simulink model "robotarm_A12"  (R2018b)
settings: Solver=FixedStepAuto  StartTime=0.0  StopTime=options.T_train  RelTol=1e-3  AbsTol=1e-6
undefined symbols (not defined in the file or in its folder): options
libraries: neural x132, simulink x2
(part 4 of 6)

== system robotarm_A12/NN/Layer 3/Delays 1 ==
  "p{3}" : Inport  PortDimensions=30
      mask Display: e = 0.06;c1 = [120 230 180]/255;c2 = ([120 230 180]+0)/(256+128);c3 = ([120 230 180]+128)/(256+128);patch([0 1 1 0],[0 0 1 1],c1);patch([0 1 1 1-e 1-e 0+e],[0 0 1 1-e 0+e 0+e],c2);patch([0 0 1 1-e 0+e 0+e],[0 1 1 1-e 1-e 0+e],c3);plot([0 1 1 0 0],[0 0 1 1 0]);
  mux : Mux  Inputs=1
      mask Display: e = 0.06;c1 = [120 150 230]/255;c2 = ([120 150 230]+0)/383;c3 = ([120 150 230]+128)/383;patch([0 1 1 0],[0 0 1 1],c1);patch([0 1 1 1-e 1-e 0+e],[0 0 1 1-e 0+e 0+e],c2);patch([0 0 1 1-e 0+e 0+e],[0 1 1 1-e 1-e 0+e],c3);plot([0 1 1 0 0],[0 0 1 1 0]);disp('Mux')
  "pd{3,2}" : Outport
      mask Display: e = 0.06;c1 = [120 230 180]/255;c2 = ([120 230 180]+0)/(256+128);c3 = ([120 230 180]+128)/(256+128);patch([0 1 1 0],[0 0 1 1],c1);patch([0 1 1 1-e 1-e 0+e],[0 0 1 1-e 0+e 0+e],c2);patch([0 0 1 1-e 0+e 0+e],[0 1 1 1-e 1-e 0+e],c3);plot([0 1 1 0 0],[0 0 1 1 0]);
  wires:
  "p{3}"/1 -> mux/1
  mux/1 -> "pd{3,2}"/1

== system robotarm_A12/NN/Layer 3/LW{3,2} ==
  "ad{3,2}" : Inport  PortDimensions=30
      mask Display: e = 0.06;c1 = [120 230 180]/255;c2 = ([120 230 180]+0)/(256+128);c3 = ([120 230 180]+128)/(256+128);patch([0 1 1 0],[0 0 1 1],c1);patch([0 1 1 1-e 1-e 0+e],[0 0 1 1-e 0+e 0+e],c2);patch([0 0 1 1-e 0+e 0+e],[0 1 1 1-e 1-e 0+e],c3);plot([0 1 1 0 0],[0 0 1 1 0]);
  "IW{3,2}(1,:)'" : Constant  Value=[0.08496298704789607969534159792601712979376316070556640625;-0.06571469853874510602675940162953338585793972015380859375;-0.06846511358825002613315291455364786088466644287109375;0.300185617440082042062243772306828759610652923583984375;-0.410231759793883654641177827215869911015033721923828125;0.37305928113203290497068564945948310196399688720703125;-0.07320623086006060320496402482604025863111019134521484375;-0.024035517098980795080986894163288525305688381195068359375;0.62376946416852285803855693302466534078121185302734375;-0.058496730913723864186959389144249144010245800018310546875;0.1466482435602333433966038001017295755445957183837890625;0.02717250980702633211816277025718591175973415374755859375;0.1705811087576470652660276527967653237283229827880859375;0.31787035680577913066002793129882775247097015380859375;-0.00835479514752205353056435654934830381534993648529052734375;0.130134459298079818712068345121224410831928253173828125;-0.1101039048182945456755277291449601761996746063232421875;-0.0571349657873238270244797831765026785433292388916015625;-0.9383620731269541881403029037755914032459259033203125;0.32545314107737366438044546157470904290676116943359375;0.133304812929548821553993320776498876512050628662109375;-0.07800643814758922989227585276239551603794097900390625;-0.6488454766229592163284678463242016732692718505859375;0.1464863330460078050254679737918195314705371856689453125;-0.29846155068246960073707896299310959875583648681640625;0.086746717271678430716264074362698011100292205810546875;-0.165613474325090714867059205062105320394039154052734375;-0.437697895520290203297264497450669296085834503173828125;-0.322682170936909706870920899746124632656574249267578125;0.29576110374639508204808180380496196448802947998046875]
      mask Display: e = 0.06;c1 = [120 150 230]/255;c2 = ([120 150 230]+0)/383;c3 = ([120 150 230]+128)/383;patch([0 1 1 0],[0 0 1 1],c1);patch([0 1 1 1-e 1-e 0+e],[0 0 1 1-e 0+e 0+e],c2);patch([0 0 1 1-e 0+e 0+e],[0 1 1 1-e 1-e 0+e],c3);plot([0 1 1 0 0],[0 0 1 1 0]);disp('weights');
  Mux : Mux  Inputs=1
      mask Display: e = 0.06;c1 = [120 150 230]/255;c2 = ([120 150 230]+0)/383;c3 = ([120 150 230]+128)/383;patch([0 1 1 0],[0 0 1 1],c1);patch([0 1 1 1-e 1-e 0+e],[0 0 1 1-e 0+e 0+e],c2);patch([0 0 1 1-e 0+e 0+e],[0 1 1 1-e 1-e 0+e],c3);plot([0 1 1 0 0],[0 0 1 1 0]);disp('Mux');
  dotprod1 : neural/Weight Functions/dotprod
  "lz{3,2}" : Outport
      mask Display: e = 0.06;c1 = [120 230 180]/255;c2 = ([120 230 180]+0)/(256+128);c3 = ([120 230 180]+128)/(256+128);patch([0 1 1 0],[0 0 1 1],c1);patch([0 1 1 1-e 1-e 0+e],[0 0 1 1-e 0+e 0+e],c2);patch([0 0 1 1-e 0+e 0+e],[0 1 1 1-e 1-e 0+e],c3);plot([0 1 1 0 0],[0 0 1 1 0]);
  wires:
  "IW{3,2}(1,:)'"/1 -> dotprod1/1
  "ad{3,2}"/1 -> dotprod1/2
  dotprod1/1 -> Mux/1
  Mux/1 -> "lz{3,2}"/1

== system robotarm_A12/NN_cex_1/Layer 1/Delays 1 ==
  "p{1}" : Inport  PortDimensions=10
      mask Display: e = 0.06;c1 = [120 230 180]/255;c2 = ([120 230 180]+0)/(256+128);c3 = ([120 230 180]+128)/(256+128);patch([0 1 1 0],[0 0 1 1],c1);patch([0 1 1 1-e 1-e 0+e],[0 0 1 1-e 0+e 0+e],c2);patch([0 0 1 1-e 0+e 0+e],[0 1 1 1-e 1-e 0+e],c3);plot([0 1 1 0 0],[0 0 1 1 0]);
  mux : Mux  Inputs=1
      mask Display: e = 0.06;c1 = [120 150 230]/255;c2 = ([120 150 230]+0)/383;c3 = ([120 150 230]+128)/383;patch([0 1 1 0],[0 0 1 1],c1);patch([0 1 1 1-e 1-e 0+e],[0 0 1 1-e 0+e 0+e],c2);patch([0 0 1 1-e 0+e 0+e],[0 1 1 1-e 1-e 0+e],c3);plot([0 1 1 0 0],[0 0 1 1 0]);disp('Mux')
  "pd{1,1}" : Outport
      mask Display: e = 0.06;c1 = [120 230 180]/255;c2 = ([120 230 180]+0)/(256+128);c3 = ([120 230 180]+128)/(256+128);patch([0 1 1 0],[0 0 1 1],c1);patch([0 1 1 1-e 1-e 0+e],[0 0 1 1-e 0+e 0+e],c2);patch([0 0 1 1-e 0+e 0+e],[0 1 1 1-e 1-e 0+e],c3);plot([0 1 1 0 0],[0 0 1 1 0]);
  wires:
  "p{1}"/1 -> mux/1
  mux/1 -> "pd{1,1}"/1

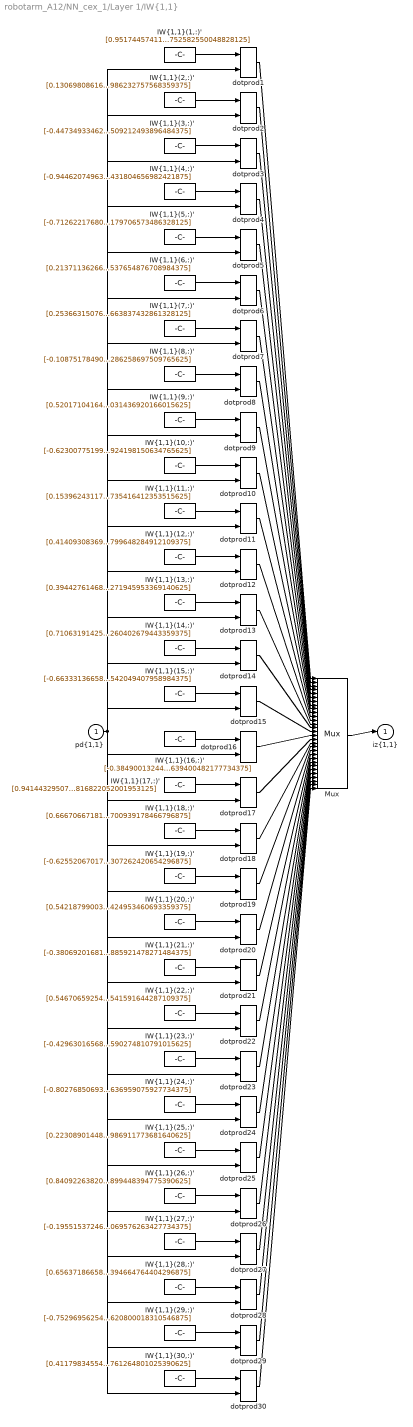
== system robotarm_A12/NN_cex_1/Layer 1/IW{1,1} ==
  "pd{1,1}" : Inport  PortDimensions=10
      mask Display: e = 0.06;c1 = [120 230 180]/255;c2 = ([120 230 180]+0)/(256+128);c3 = ([120 230 180]+128)/(256+128);patch([0 1 1 0],[0 0 1 1],c1);patch([0 1 1 1-e 1-e 0+e],[0 0 1 1-e 0+e 0+e],c2);patch([0 0 1 1-e 0+e 0+e],[0 1 1 1-e 1-e 0+e],c3);plot([0 1 1 0 0],[0 0 1 1 0]);
  "IW{1,1}(1,:)'" : Constant  Value=[0.95174457411673751838776524891727603971958160400390625;-0.1217696827207606080634150202968157827854156494140625;-0.3515402442307336006166451625176705420017242431640625;-0.1259480441304231257415580103042884729802608489990234375;0.80008138770185077692786990155582316219806671142578125;0.74164545184093244589718096904107369482517242431640625;-0.406940495434214455361399132016231305897235870361328125;0.70915830977854599215248754262574948370456695556640625;-0.416282474324658924302866580546833574771881103515625;0.2759902705292305302720023973961360752582550048828125]
      mask Display: e = 0.06;c1 = [120 150 230]/255;c2 = ([120 150 230]+0)/383;c3 = ([120 150 230]+128)/383;patch([0 1 1 0],[0 0 1 1],c1);patch([0 1 1 1-e 1-e 0+e],[0 0 1 1-e 0+e 0+e],c2);patch([0 0 1 1-e 0+e 0+e],[0 1 1 1-e 1-e 0+e],c3);plot([0 1 1 0 0],[0 0 1 1 0]);disp('Weights');
  "IW{1,1}(10,:)'" : Constant  Value=[-0.623007751998844394591969830798916518688201904296875;-0.229780936649281730677074619961786083877086639404296875;0.7291435892727637924082273457315750420093536376953125;-0.35662187514995746795420927810482680797576904296875;0.42812272845337473459181865109712816774845123291015625;-0.11093840865894664948765324652413255535066127777099609375;0.52830304957231655205163178834482096135616302490234375;-0.252988660476427706935709238678100518882274627685546875;-0.6660480731444315960487756456132046878337860107421875;-0.58246326337977072373774944935576058924198150634765625]
      mask Display: e = 0.06;c1 = [120 150 230]/255;c2 = ([120 150 230]+0)/383;c3 = ([120 150 230]+128)/383;patch([0 1 1 0],[0 0 1 1],c1);patch([0 1 1 1-e 1-e 0+e],[0 0 1 1-e 0+e 0+e],c2);patch([0 0 1 1-e 0+e 0+e],[0 1 1 1-e 1-e 0+e],c3);plot([0 1 1 0 0],[0 0 1 1 0]);disp('Weights');
  "IW{1,1}(11,:)'" : Constant  Value=[0.1539624311750474039417468929968890734016895294189453125;0.7416396906165083624529188455198891460895538330078125;-0.60468007765930387176211979749496094882488250732421875;-0.245839274571849342176932395886979065835475921630859375;0.40883791938954894273905438240035437047481536865234375;-0.94945320706745750527488780790008604526519775390625;0.6006005707831933992935091737308539450168609619140625;0.56612393711479425117971686631790362298488616943359375;-0.184880190142234390737741023258422501385211944580078125;-0.57581437728133677556030534105957485735416412353515625]
      mask Display: e = 0.06;c1 = [120 150 230]/255;c2 = ([120 150 230]+0)/383;c3 = ([120 150 230]+128)/383;patch([0 1 1 0],[0 0 1 1],c1);patch([0 1 1 1-e 1-e 0+e],[0 0 1 1-e 0+e 0+e],c2);patch([0 0 1 1-e 0+e 0+e],[0 1 1 1-e 1-e 0+e],c3);plot([0 1 1 0 0],[0 0 1 1 0]);disp('Weights');
  "IW{1,1}(12,:)'" : Constant  Value=[0.41409308369847874775615537146222777664661407470703125;0.1875357709384890825266012370775570161640644073486328125;0.768771241957419082524438636028207838535308837890625;0.0114774948924922792770075830048881471157073974609375;0.6372438759351302106637149336165748536586761474609375;0.411372095929997627639096435814280994236469268798828125;-0.171189467147416729542186430990113876760005950927734375;0.3941923804447144963347682278254069387912750244140625;-0.78954036993725240645147778195678256452083587646484375;0.6864763546809589112029925672686658799648284912109375]
      mask Display: e = 0.06;c1 = [120 150 230]/255;c2 = ([120 150 230]+0)/383;c3 = ([120 150 230]+128)/383;patch([0 1 1 0],[0 0 1 1],c1);patch([0 1 1 1-e 1-e 0+e],[0 0 1 1-e 0+e 0+e],c2);patch([0 0 1 1-e 0+e 0+e],[0 1 1 1-e 1-e 0+e],c3);plot([0 1 1 0 0],[0 0 1 1 0]);disp('Weights');
  "IW{1,1}(13,:)'" : Constant  Value=[0.394427614683170724152461161793326027691364288330078125;0.53940731643208461587590818453463725745677947998046875;-1.2160364242706951376504775907960720360279083251953125;-0.03782517365620241545087765189236961305141448974609375;0.28938754106922548459124300279654562473297119140625;0.41714626880523508756226647165021859109401702880859375;0.00343580126263719025370146908926471951417624950408935546875;-0.73889468146552450544817247646278701722621917724609375;0.83357367460742748388469181008986197412014007568359375;0.0303053862099035044297412611058462061919271945953369140625]
      mask Display: e = 0.06;c1 = [120 150 230]/255;c2 = ([120 150 230]+0)/383;c3 = ([120 150 230]+128)/383;patch([0 1 1 0],[0 0 1 1],c1);patch([0 1 1 1-e 1-e 0+e],[0 0 1 1-e 0+e 0+e],c2);patch([0 0 1 1-e 0+e 0+e],[0 1 1 1-e 1-e 0+e],c3);plot([0 1 1 0 0],[0 0 1 1 0]);disp('Weights');
  "IW{1,1}(14,:)'" : Constant  Value=[0.71063191425381921906279103495762683451175689697265625;0.187637820172291636122707814138266257941722869873046875;-0.265860645834559428113408330318634398281574249267578125;-1.0317094380765958749890387480263598263263702392578125;-0.72702378170373693766492806389578618109226226806640625;0.2085283569264141656507405286902212537825107574462890625;-0.469377781256357817785129782350850291550159454345703125;0.990661527702205280121461328235454857349395751953125;-0.36777067572498689518312176005565561354160308837890625;0.159778158397644032273632319629541598260402679443359375]
      mask Display: e = 0.06;c1 = [120 150 230]/255;c2 = ([120 150 230]+0)/383;c3 = ([120 150 230]+128)/383;patch([0 1 1 0],[0 0 1 1],c1);patch([0 1 1 1-e 1-e 0+e],[0 0 1 1-e 0+e 0+e],c2);patch([0 0 1 1-e 0+e 0+e],[0 1 1 1-e 1-e 0+e],c3);plot([0 1 1 0 0],[0 0 1 1 0]);disp('Weights');
  "IW{1,1}(15,:)'" : Constant  Value=[-0.66333136658032454402444955121609382331371307373046875;0.0283706812461598512076221823008381761610507965087890625;0.947155627404870248398083276697434484958648681640625;0.11165785886550409766737601557906600646674633026123046875;0.00079959436163776730077668020157943828962743282318115234375;-0.8754131708892221030993141539511270821094512939453125;0.67663448294062200627507763783796690404415130615234375;-0.13894066218460665584899516034056432545185089111328125;-0.51722680556951494690309800716931931674480438232421875;-0.70023846525171451471436512292711995542049407958984375]
      mask Display: e = 0.06;c1 = [120 150 230]/255;c2 = ([120 150 230]+0)/383;c3 = ([120 150 230]+128)/383;patch([0 1 1 0],[0 0 1 1],c1);patch([0 1 1 1-e 1-e 0+e],[0 0 1 1-e 0+e 0+e],c2);patch([0 0 1 1-e 0+e 0+e],[0 1 1 1-e 1-e 0+e],c3);plot([0 1 1 0 0],[0 0 1 1 0]);disp('Weights');
  "IW{1,1}(16,:)'" : Constant  Value=[-0.38490013244770293621144219287089072167873382568359375;0.9810023910127154689320150282583199441432952880859375;0.251112718851861094204735991297638975083827972412109375;-0.263318959585589540406402875305502675473690032958984375;0.2316317856842861344635053910678834654390811920166015625;-0.57991803645792561194838299343246035277843475341796875;0.102099604854992975777605579423834569752216339111328125;0.0757096886541124280967096638050861656665802001953125;0.94700532225513978090702948975376784801483154296875;0.2264528826197016453392052426352165639400482177734375]
      mask Display: e = 0.06;c1 = [120 150 230]/255;c2 = ([120 150 230]+0)/383;c3 = ([120 150 230]+128)/383;patch([0 1 1 0],[0 0 1 1],c1);patch([0 1 1 1-e 1-e 0+e],[0 0 1 1-e 0+e 0+e],c2);patch([0 0 1 1-e 0+e 0+e],[0 1 1 1-e 1-e 0+e],c3);plot([0 1 1 0 0],[0 0 1 1 0]);disp('Weights');
  "IW{1,1}(17,:)'" : Constant  Value=[0.94144329507807034129740486605442129075527191162109375;-0.73965966230873103626208830974064767360687255859375;-0.07130712020036622522667357770842500030994415283203125;-0.2208399818406310277651982687530107796192169189453125;-0.277789871801359999903269226706470362842082977294921875;-0.359897691306751088546889150165952742099761962890625;0.9601340515891567672923656573402695357799530029296875;-0.369316870611459402429233023212873376905918121337890625;-0.74597811794454160772005479884683154523372650146484375;-0.78633224578286420314299220990506000816822052001953125]
      mask Display: e = 0.06;c1 = [120 150 230]/255;c2 = ([120 150 230]+0)/383;c3 = ([120 150 230]+128)/383;patch([0 1 1 0],[0 0 1 1],c1);patch([0 1 1 1-e 1-e 0+e],[0 0 1 1-e 0+e 0+e],c2);patch([0 0 1 1-e 0+e 0+e],[0 1 1 1-e 1-e 0+e],c3);plot([0 1 1 0 0],[0 0 1 1 0]);disp('Weights');
  "IW{1,1}(18,:)'" : Constant  Value=[0.6667066718183065621161631497670896351337432861328125;-0.5473546682509569105690161450183950364589691162109375;0.0233489465669737931985405765544783207587897777557373046875;0.7702377271502787170476267419871874153614044189453125;-0.55090505365841468954357651455211453139781951904296875;0.3660903597738933701322139313560910522937774658203125;0.7190503595666071223746484974981285631656646728515625;-0.79804653873549558085187527467496693134307861328125;0.51570704016299095950870423621381632983684539794921875;-0.08422010419312513096468109097259002737700939178466796875]
      mask Display: e = 0.06;c1 = [120 150 230]/255;c2 = ([120 150 230]+0)/383;c3 = ([120 150 230]+128)/383;patch([0 1 1 0],[0 0 1 1],c1);patch([0 1 1 1-e 1-e 0+e],[0 0 1 1-e 0+e 0+e],c2);patch([0 0 1 1-e 0+e 0+e],[0 1 1 1-e 1-e 0+e],c3);plot([0 1 1 0 0],[0 0 1 1 0]);disp('Weights');
  "IW{1,1}(19,:)'" : Constant  Value=[-0.6255206701708557748276007259846664965152740478515625;-0.374719888708542392397049525243346579372882843017578125;0.9966336869345850946189102614880539476871490478515625;-0.3122926507044614385932845834759064018726348876953125;0.290043586731720093307984598141047172248363494873046875;0.613414969810574195463459545862860977649688720703125;-0.8267832172506774934817030953126959502696990966796875;0.1475166835789429864433941474999301135540008544921875;0.375160016384135708289448984942282550036907196044921875;0.8298608043035986536750669984030537307262420654296875]
      mask Display: e = 0.06;c1 = [120 150 230]/255;c2 = ([120 150 230]+0)/383;c3 = ([120 150 230]+128)/383;patch([0 1 1 0],[0 0 1 1],c1);patch([0 1 1 1-e 1-e 0+e],[0 0 1 1-e 0+e 0+e],c2);patch([0 0 1 1-e 0+e 0+e],[0 1 1 1-e 1-e 0+e],c3);plot([0 1 1 0 0],[0 0 1 1 0]);disp('Weights');
  "IW{1,1}(2,:)'" : Constant  Value=[0.1306980861606092947369006651570089161396026611328125;0.95496961844291583521027177994255907833576202392578125;0.07114737585953608001165804353149724192917346954345703125;-0.9014571916909137616613634236273355782032012939453125;-0.72337058173384860548793540147016756236553192138671875;0.8099059820216663041492211050353944301605224609375;-0.71090354732238625334872494931914843618869781494140625;0.264037695535799754598116351189673878252506256103515625;-0.46725463080554774375485749260406009852886199951171875;0.474530247970752439012898094006231985986232757568359375]
      mask Display: e = 0.06;c1 = [120 150 230]/255;c2 = ([120 150 230]+0)/383;c3 = ([120 150 230]+128)/383;patch([0 1 1 0],[0 0 1 1],c1);patch([0 1 1 1-e 1-e 0+e],[0 0 1 1-e 0+e 0+e],c2);patch([0 0 1 1-e 0+e 0+e],[0 1 1 1-e 1-e 0+e],c3);plot([0 1 1 0 0],[0 0 1 1 0]);disp('Weights');
  "IW{1,1}(20,:)'" : Constant  Value=[0.54218799003624418286761965646292082965373992919921875;-1.0245248233144270688654842160758562386035919189453125;0.9164331846045523644050945222261361777782440185546875;0.753343654544192720123874096316285431385040283203125;0.07592826697309439099026207031783997081220149993896484375;0.3176901400103206984937287415959872305393218994140625;0.176133734619415671662778777317726053297519683837890625;0.42562796066195096589268587194965220987796783447265625;0.456211541935506448286474778797128237783908843994140625;0.557171419964075820274729267111979424953460693359375]
      mask Display: e = 0.06;c1 = [120 150 230]/255;c2 = ([120 150 230]+0)/383;c3 = ([120 150 230]+128)/383;patch([0 1 1 0],[0 0 1 1],c1);patch([0 1 1 1-e 1-e 0+e],[0 0 1 1-e 0+e 0+e],c2);patch([0 0 1 1-e 0+e 0+e],[0 1 1 1-e 1-e 0+e],c3);plot([0 1 1 0 0],[0 0 1 1 0]);disp('Weights');
  "IW{1,1}(21,:)'" : Constant  Value=[-0.3806920168155050188119048470980487763881683349609375;0.56863128261064554980208640699856914579868316650390625;0.060980204521940362116794176472467370331287384033203125;0.7878789891283528579180028827977366745471954345703125;0.90247671351418612406547481441521085798740386962890625;-0.01024721592672982357907773831584563595242798328399658203125;0.76907463502263329058195040488499216735363006591796875;0.1458937326053030003603083741836599074304103851318359375;0.66018927714307362730750128321233205497264862060546875;-0.606270977882802153402508338331244885921478271484375]
      mask Display: e = 0.06;c1 = [120 150 230]/255;c2 = ([120 150 230]+0)/383;c3 = ([120 150 230]+128)/383;patch([0 1 1 0],[0 0 1 1],c1);patch([0 1 1 1-e 1-e 0+e],[0 0 1 1-e 0+e 0+e],c2);patch([0 0 1 1-e 0+e 0+e],[0 1 1 1-e 1-e 0+e],c3);plot([0 1 1 0 0],[0 0 1 1 0]);disp('Weights');
  "IW{1,1}(22,:)'" : Constant  Value=[0.54670659254256526171644736677990294992923736572265625;-0.82515026660895129939632397508830763399600982666015625;-0.70786451044767717544203833313076756894588470458984375;0.42151771314947106272796872872277162969112396240234375;-0.87171495474021887250870577190653420984745025634765625;1.055883044828184846863905477221123874187469482421875;0.0942092134405958792076063446074840612709522247314453125;0.2147213331631441513014380007007275708019733428955078125;-0.11783780791913199548215374079518369399011135101318359375;0.1525560191211824123680429465821362100541591644287109375]
      mask Display: e = 0.06;c1 = [120 150 230]/255;c2 = ([120 150 230]+0)/383;c3 = ([120 150 230]+128)/383;patch([0 1 1 0],[0 0 1 1],c1);patch([0 1 1 1-e 1-e 0+e],[0 0 1 1-e 0+e 0+e],c2);patch([0 0 1 1-e 0+e 0+e],[0 1 1 1-e 1-e 0+e],c3);plot([0 1 1 0 0],[0 0 1 1 0]);disp('Weights');
  "IW{1,1}(23,:)'" : Constant  Value=[-0.429630165689424192709822136748698540031909942626953125;0.155084445770670098507792999953380785882472991943359375;-0.9095263878210582131345063316985033452510833740234375;0.7505049233271472441941796205355785787105560302734375;0.4178919102309428534880453298683278262615203857421875;0.40308685973617330855489626628695987164974212646484375;0.764317545750285542993651688448153436183929443359375;-0.0164411878385180044992441850126851932145655155181884765625;-0.632931394122257184875479651964269578456878662109375;-0.66019443942390465540626109941513277590274810791015625]
      mask Display: e = 0.06;c1 = [120 150 230]/255;c2 = ([120 150 230]+0)/383;c3 = ([120 150 230]+128)/383;patch([0 1 1 0],[0 0 1 1],c1);patch([0 1 1 1-e 1-e 0+e],[0 0 1 1-e 0+e 0+e],c2);patch([0 0 1 1-e 0+e 0+e],[0 1 1 1-e 1-e 0+e],c3);plot([0 1 1 0 0],[0 0 1 1 0]);disp('Weights');
  "IW{1,1}(24,:)'" : Constant  Value=[-0.8027685069395691375149226587382145226001739501953125;0.54345797507239235191178750028484500944614410400390625;-1.0587767969113899280131363411783240735530853271484375;-0.2117637152008174095119130697639775462448596954345703125;-0.9420896446882718322513028397224843502044677734375;-0.200844407227330934428977116112946532666683197021484375;0.329009011982244914396034118908573873341083526611328125;-0.25333913565001997536541011868393979966640472412109375;0.1520572383388081594279839237060514278709888458251953125;-0.1990589940299736237960814833058975636959075927734375]
      mask Display: e = 0.06;c1 = [120 150 230]/255;c2 = ([120 150 230]+0)/383;c3 = ([120 150 230]+128)/383;patch([0 1 1 0],[0 0 1 1],c1);patch([0 1 1 1-e 1-e 0+e],[0 0 1 1-e 0+e 0+e],c2);patch([0 0 1 1-e 0+e 0+e],[0 1 1 1-e 1-e 0+e],c3);plot([0 1 1 0 0],[0 0 1 1 0]);disp('Weights');
  "IW{1,1}(25,:)'" : Constant  Value=[0.2230890144841241873319148680820944719016551971435546875;0.478806718750225901448658305525896139442920684814453125;0.775923306728495187911676111980341374874114990234375;0.2207830370020641141959316655629663728177547454833984375;0.8995007162111170462281961590633727610111236572265625;1.0189648959053918542139172132010571658611297607421875;-0.7753993971354027348041881850804202258586883544921875;-0.439551628286339590712117342263809405267238616943359375;0.382946465539386660115184213282191194593906402587890625;0.09517768290046137169557738388903089798986911773681640625]
      mask Display: e = 0.06;c1 = [120 150 230]/255;c2 = ([120 150 230]+0)/383;c3 = ([120 150 230]+128)/383;patch([0 1 1 0],[0 0 1 1],c1);patch([0 1 1 1-e 1-e 0+e],[0 0 1 1-e 0+e 0+e],c2);patch([0 0 1 1-e 0+e 0+e],[0 1 1 1-e 1-e 0+e],c3);plot([0 1 1 0 0],[0 0 1 1 0]);disp('Weights');
  "IW{1,1}(26,:)'" : Constant  Value=[0.84092263820767854110016514823655597865581512451171875;-0.57090397085884159178448271632078103721141815185546875;-0.2460686743491804218120222458310308866202831268310546875;-0.6051406275744668494809275216539390385150909423828125;-0.166803359359675773543330024040187709033489227294921875;0.290888359900464299467870432636118493974208831787109375;0.49256982629871359780082684665103442966938018798828125;-0.360211590216723387403163769704406149685382843017578125;0.56054316498180389860550576486275531351566314697265625;0.86333408939697964257220519357360899448394775390625]
      mask Display: e = 0.06;c1 = [120 150 230]/255;c2 = ([120 150 230]+0)/383;c3 = ([120 150 230]+128)/383;patch([0 1 1 0],[0 0 1 1],c1);patch([0 1 1 1-e 1-e 0+e],[0 0 1 1-e 0+e 0+e],c2);patch([0 0 1 1-e 0+e 0+e],[0 1 1 1-e 1-e 0+e],c3);plot([0 1 1 0 0],[0 0 1 1 0]);disp('Weights');
  "IW{1,1}(27,:)'" : Constant  Value=[-0.195515372466835035680787768797017633914947509765625;0.7173315931382455712395085356547497212886810302734375;-0.2402386867008234616616135781441698782145977020263671875;0.49013000562788278102743788622319698333740234375;-0.23598130298790531700348083177232183516025543212890625;0.21408569882975225784349504465353675186634063720703125;0.91983061449868730452550380505272187292575836181640625;-0.6196964740371939672769485696335323154926300048828125;-0.85238921614023421824413162539713084697723388671875;-0.481091399081892967526385973542346619069576263427734375]
      mask Display: e = 0.06;c1 = [120 150 230]/255;c2 = ([120 150 230]+0)/383;c3 = ([120 150 230]+128)/383;patch([0 1 1 0],[0 0 1 1],c1);patch([0 1 1 1-e 1-e 0+e],[0 0 1 1-e 0+e 0+e],c2);patch([0 0 1 1-e 0+e 0+e],[0 1 1 1-e 1-e 0+e],c3);plot([0 1 1 0 0],[0 0 1 1 0]);disp('Weights');
  "IW{1,1}(28,:)'" : Constant  Value=[0.6563718665879030300658314445172436535358428955078125;0.3681304659076471974543665055534802377223968505859375;0.2643473592544147710015067787026055157184600830078125;0.009756369109199837519330600343892001546919345855712890625;-0.93239914053506811608684756720322184264659881591796875;1.2291875398967615495848804130218923091888427734375;-0.24105674116655517735807734425179660320281982421875;-0.53276237084788158338000130243017338216304779052734375;0.050333288412835262837230487775741494260728359222412109375;-0.42764414470663669742833690179395489394664764404296875]
      mask Display: e = 0.06;c1 = [120 150 230]/255;c2 = ([120 150 230]+0)/383;c3 = ([120 150 230]+128)/383;patch([0 1 1 0],[0 0 1 1],c1);patch([0 1 1 1-e 1-e 0+e],[0 0 1 1-e 0+e 0+e],c2);patch([0 0 1 1-e 0+e 0+e],[0 1 1 1-e 1-e 0+e],c3);plot([0 1 1 0 0],[0 0 1 1 0]);disp('Weights');
  "IW{1,1}(29,:)'" : Constant  Value=[-0.752969562544694159811342615284956991672515869140625;-0.0690264886534393828920741498222923837602138519287109375;0.061723299889448642041589465634388034231960773468017578125;-0.8258187418584437278212817545863799750804901123046875;-0.54528318676246190221945653320290148258209228515625;0.66651865242649022125220881207496859133243560791015625;0.240205888676898238198731405645958147943019866943359375;-0.61930024833245023163641462815576232969760894775390625;0.35645987741214335553507908116444014012813568115234375;0.6761211152102741817060405082884244620800018310546875]
      mask Display: e = 0.06;c1 = [120 150 230]/255;c2 = ([120 150 230]+0)/383;c3 = ([120 150 230]+128)/383;patch([0 1 1 0],[0 0 1 1],c1);patch([0 1 1 1-e 1-e 0+e],[0 0 1 1-e 0+e 0+e],c2);patch([0 0 1 1-e 0+e 0+e],[0 1 1 1-e 1-e 0+e],c3);plot([0 1 1 0 0],[0 0 1 1 0]);disp('Weights');
  "IW{1,1}(3,:)'" : Constant  Value=[-0.44734933462095261003099722074694000184535980224609375;0.281022309728365449199571912686224095523357391357421875;-0.43887247168385312701133216251037083566188812255859375;-0.8198232524992612457737095610355027019977569580078125;0.7199127282938206917606294155120849609375;0.9016884924018981894988655767519958317279815673828125;-0.247923906546288208563311172838439233601093292236328125;-0.395012912494521639672484525362960994243621826171875;0.3982470900420567172517394283204339444637298583984375;0.50457516186721862450070830163895152509212493896484375]
      mask Display: e = 0.06;c1 = [120 150 230]/255;c2 = ([120 150 230]+0)/383;c3 = ([120 150 230]+128)/383;patch([0 1 1 0],[0 0 1 1],c1);patch([0 1 1 1-e 1-e 0+e],[0 0 1 1-e 0+e 0+e],c2);patch([0 0 1 1-e 0+e 0+e],[0 1 1 1-e 1-e 0+e],c3);plot([0 1 1 0 0],[0 0 1 1 0]);disp('Weights');
  "IW{1,1}(30,:)'" : Constant  Value=[0.411798345545783262000583135886699892580509185791015625;0.63927833386715093855201530459453351795673370361328125;-0.6444806899967769897585867511224932968616485595703125;-0.320945860388249515349201601566164754331111907958984375;-0.362895848682063870693781382215092889964580535888671875;-0.67025309086907025601931309211067855358123779296875;0.9579691680816624366201494922279380261898040771484375;-0.85798240549095006191038237375323660671710968017578125;-0.411104600059531255507039304575300775468349456787109375;-0.466387818422207056645589773324900306761264801025390625]
      mask Display: e = 0.06;c1 = [120 150 230]/255;c2 = ([120 150 230]+0)/383;c3 = ([120 150 230]+128)/383;patch([0 1 1 0],[0 0 1 1],c1);patch([0 1 1 1-e 1-e 0+e],[0 0 1 1-e 0+e 0+e],c2);patch([0 0 1 1-e 0+e 0+e],[0 1 1 1-e 1-e 0+e],c3);plot([0 1 1 0 0],[0 0 1 1 0]);disp('Weights');
  "IW{1,1}(4,:)'" : Constant  Value=[-0.944620749630243228267545418930239975452423095703125;0.391164777450933254243636838509701192378997802734375;-0.373189825015530718399503484761225990951061248779296875;-0.480306119501472006394493519110255874693393707275390625;-0.32205016552848675370768205539206974208354949951171875;-0.6057818195193924726282830306445248425006866455078125;-0.60802051960651903872445700471871532499790191650390625;-0.449251332234870182080754830167279578745365142822265625;-0.75732058115572320478037227076129056513309478759765625;0.65699739705545645573891988533432595431804656982421875]
      mask Display: e = 0.06;c1 = [120 150 230]/255;c2 = ([120 150 230]+0)/383;c3 = ([120 150 230]+128)/383;patch([0 1 1 0],[0 0 1 1],c1);patch([0 1 1 1-e 1-e 0+e],[0 0 1 1-e 0+e 0+e],c2);patch([0 0 1 1-e 0+e 0+e],[0 1 1 1-e 1-e 0+e],c3);plot([0 1 1 0 0],[0 0 1 1 0]);disp('Weights');
  "IW{1,1}(5,:)'" : Constant  Value=[-0.71262217680880668435605684862821362912654876708984375;0.6963802530691431957876602609758265316486358642578125;0.589940040498455164907909420435316860675811767578125;0.58633236455164183809074529563076794147491455078125;0.8274084564087804682941396094975061714649200439453125;-0.1656711341334670406499895989327342249453067779541015625;-0.51425040539413491291753643963602371513843536376953125;0.06840672681284988565497684476213180460035800933837890625;0.70476831946459406186278329187189228832721710205078125;0.2501250149177451920223802517284639179706573486328125]
      mask Display: e = 0.06;c1 = [120 150 230]/255;c2 = ([120 150 230]+0)/383;c3 = ([120 150 230]+128)/383;patch([0 1 1 0],[0 0 1 1],c1);patch([0 1 1 1-e 1-e 0+e],[0 0 1 1-e 0+e 0+e],c2);patch([0 0 1 1-e 0+e 0+e],[0 1 1 1-e 1-e 0+e],c3);plot([0 1 1 0 0],[0 0 1 1 0]);disp('Weights');
  "IW{1,1}(6,:)'" : Constant  Value=[0.213711362668614957005530641254154033958911895751953125;0.79317037935154777184010299606597982347011566162109375;-0.88484287981779186083031163434498012065887451171875;-0.064311727026041209942519571995944716036319732666015625;-0.434297277034422835040317067978321574628353118896484375;-0.74783778020945301800992410790058784186840057373046875;-0.09291065599116861417616775042915833182632923126220703125;0.08414618770079140830375763471238315105438232421875;0.0212503578853590856245769913357435143552720546722412109375;-0.77679574980022836339088598833768628537654876708984375]
      mask Display: e = 0.06;c1 = [120 150 230]/255;c2 = ([120 150 230]+0)/383;c3 = ([120 150 230]+128)/383;patch([0 1 1 0],[0 0 1 1],c1);patch([0 1 1 1-e 1-e 0+e],[0 0 1 1-e 0+e 0+e],c2);patch([0 0 1 1-e 0+e 0+e],[0 1 1 1-e 1-e 0+e],c3);plot([0 1 1 0 0],[0 0 1 1 0]);disp('Weights');
  "IW{1,1}(7,:)'" : Constant  Value=[0.253663150762862610321235479204915463924407958984375;-0.621190039290176354569439354236237704753875732421875;0.673545164343586133526287085260264575481414794921875;0.5212910628691498349240873722010292112827301025390625;0.6341752291286208986775818630121648311614990234375;0.55776338432429373170862163533456623554229736328125;-0.53517417251864729532684350488125346601009368896484375;-0.7302343563854929442413776996545493602752685546875;-0.49275747808096082014372996127349324524402618408203125;-0.0706697469994979343699270657452871091663837432861328125]
      mask Display: e = 0.06;c1 = [120 150 230]/255;c2 = ([120 150 230]+0)/383;c3 = ([120 150 230]+128)/383;patch([0 1 1 0],[0 0 1 1],c1);patch([0 1 1 1-e 1-e 0+e],[0 0 1 1-e 0+e 0+e],c2);patch([0 0 1 1-e 0+e 0+e],[0 1 1 1-e 1-e 0+e],c3);plot([0 1 1 0 0],[0 0 1 1 0]);disp('Weights');
  "IW{1,1}(8,:)'" : Constant  Value=[-0.1087517849041293171996613864394021220505237579345703125;0.01302669343997702768034319120715736062265932559967041015625;-0.2877792446313296448323626464116387069225311279296875;-0.75553220097485118689206728959106840193271636962890625;-0.6099660416198828816192190060974098742008209228515625;-0.220764001818420541045639993171789683401584625244140625;-0.722601338827775219186833055573515594005584716796875;-0.77406809990615965677562826385837979614734649658203125;0.142333657097201193852953338137012906372547149658203125;0.45329105148377257794578554239706136286258697509765625]
      mask Display: e = 0.06;c1 = [120 150 230]/255;c2 = ([120 150 230]+0)/383;c3 = ([120 150 230]+128)/383;patch([0 1 1 0],[0 0 1 1],c1);patch([0 1 1 1-e 1-e 0+e],[0 0 1 1-e 0+e 0+e],c2);patch([0 0 1 1-e 0+e 0+e],[0 1 1 1-e 1-e 0+e],c3);plot([0 1 1 0 0],[0 0 1 1 0]);disp('Weights');
  "IW{1,1}(9,:)'" : Constant  Value=[0.52017104164383420883410735768848098814487457275390625;-0.0534751907150148586556070995357003994286060333251953125;-0.045872170547628744741164297238356084562838077545166015625;-0.5640387829424813315171149952220730483531951904296875;0.224410184451367566982327161895227618515491485595703125;0.51155203514828972988226496454444713890552520751953125;-0.19330480750684608803879882543697021901607513427734375;0.85672531104375237998027614594320766627788543701171875;0.309236574318380252890392512199468910694122314453125;-0.7181829350665991373858787483186461031436920166015625]
      mask Display: e = 0.06;c1 = [120 150 230]/255;c2 = ([120 150 230]+0)/383;c3 = ([120 150 230]+128)/383;patch([0 1 1 0],[0 0 1 1],c1);patch([0 1 1 1-e 1-e 0+e],[0 0 1 1-e 0+e 0+e],c2);patch([0 0 1 1-e 0+e 0+e],[0 1 1 1-e 1-e 0+e],c3);plot([0 1 1 0 0],[0 0 1 1 0]);disp('Weights');
  Mux : Mux  Inputs=30
      mask Display: e = 0.06;c1 = [120 150 230]/255;c2 = ([120 150 230]+0)/383;c3 = ([120 150 230]+128)/383;patch([0 1 1 0],[0 0 1 1],c1);patch([0 1 1 1-e 1-e 0+e],[0 0 1 1-e 0+e 0+e],c2);patch([0 0 1 1-e 0+e 0+e],[0 1 1 1-e 1-e 0+e],c3);plot([0 1 1 0 0],[0 0 1 1 0]);disp('Mux');
  dotprod{1..30} (30 alike) : neural/Weight Functions/dotprod
  "iz{1,1}" : Outport
      mask Display: e = 0.06;c1 = [120 230 180]/255;c2 = ([120 230 180]+0)/(256+128);c3 = ([120 230 180]+128)/(256+128);patch([0 1 1 0],[0 0 1 1],c1);patch([0 1 1 1-e 1-e 0+e],[0 0 1 1-e 0+e 0+e],c2);patch([0 0 1 1-e 0+e 0+e],[0 1 1 1-e 1-e 0+e],c3);plot([0 1 1 0 0],[0 0 1 1 0]);
  wires:
  "IW{1,1}(1,:)'"/1 -> dotprod1/1
  "pd{1,1}"/1 -> dotprod1/2, dotprod2/2, dotprod3/2, dotprod4/2, dotprod5/2, dotprod6/2, dotprod7/2, dotprod8/2, dotprod9/2, dotprod10/2, dotprod11/2, dotprod12/2, dotprod13/2, dotprod14/2, dotprod15/2, dotprod16/2, dotprod17/2, dotprod18/2, dotprod19/2, dotprod20/2, dotprod21/2, dotprod22/2, dotprod23/2, dotprod24/2, dotprod25/2, dotprod26/2, dotprod27/2, dotprod28/2, dotprod29/2, dotprod30/2
  dotprod1/1 -> Mux/1
  "IW{1,1}(2,:)'"/1 -> dotprod2/1
  dotprod2/1 -> Mux/2
  "IW{1,1}(3,:)'"/1 -> dotprod3/1
  dotprod3/1 -> Mux/3
  "IW{1,1}(4,:)'"/1 -> dotprod4/1
  dotprod4/1 -> Mux/4
  "IW{1,1}(5,:)'"/1 -> dotprod5/1
  dotprod5/1 -> Mux/5
  "IW{1,1}(6,:)'"/1 -> dotprod6/1
  dotprod6/1 -> Mux/6
  "IW{1,1}(7,:)'"/1 -> dotprod7/1
  dotprod7/1 -> Mux/7
  "IW{1,1}(8,:)'"/1 -> dotprod8/1
  dotprod8/1 -> Mux/8
  "IW{1,1}(9,:)'"/1 -> dotprod9/1
  dotprod9/1 -> Mux/9
  "IW{1,1}(10,:)'"/1 -> dotprod10/1
  dotprod10/1 -> Mux/10
  "IW{1,1}(11,:)'"/1 -> dotprod11/1
  dotprod11/1 -> Mux/11
  "IW{1,1}(12,:)'"/1 -> dotprod12/1
  dotprod12/1 -> Mux/12
  "IW{1,1}(13,:)'"/1 -> dotprod13/1
  dotprod13/1 -> Mux/13
  "IW{1,1}(14,:)'"/1 -> dotprod14/1
  dotprod14/1 -> Mux/14
  "IW{1,1}(15,:)'"/1 -> dotprod15/1
  dotprod15/1 -> Mux/15
  "IW{1,1}(16,:)'"/1 -> dotprod16/1
  dotprod16/1 -> Mux/16
  "IW{1,1}(17,:)'"/1 -> dotprod17/1
  dotprod17/1 -> Mux/17
  "IW{1,1}(18,:)'"/1 -> dotprod18/1
  dotprod18/1 -> Mux/18
  "IW{1,1}(19,:)'"/1 -> dotprod19/1
  dotprod19/1 -> Mux/19
  "IW{1,1}(20,:)'"/1 -> dotprod20/1
  dotprod20/1 -> Mux/20
  "IW{1,1}(21,:)'"/1 -> dotprod21/1
  dotprod21/1 -> Mux/21
  "IW{1,1}(22,:)'"/1 -> dotprod22/1
  dotprod22/1 -> Mux/22
  "IW{1,1}(23,:)'"/1 -> dotprod23/1
  dotprod23/1 -> Mux/23
  "IW{1,1}(24,:)'"/1 -> dotprod24/1
  dotprod24/1 -> Mux/24
  "IW{1,1}(25,:)'"/1 -> dotprod25/1
  dotprod25/1 -> Mux/25
  "IW{1,1}(26,:)'"/1 -> dotprod26/1
  dotprod26/1 -> Mux/26
  "IW{1,1}(27,:)'"/1 -> dotprod27/1
  dotprod27/1 -> Mux/27
  "IW{1,1}(28,:)'"/1 -> dotprod28/1
  dotprod28/1 -> Mux/28
  "IW{1,1}(29,:)'"/1 -> dotprod29/1
  dotprod29/1 -> Mux/29
  "IW{1,1}(30,:)'"/1 -> dotprod30/1
  dotprod30/1 -> Mux/30
  Mux/1 -> "iz{1,1}"/1

== system robotarm_A12/NN_cex_1/Layer 2/Delays 1 ==
  "p{2}" : Inport  PortDimensions=30
      mask Display: e = 0.06;c1 = [120 230 180]/255;c2 = ([120 230 180]+0)/(256+128);c3 = ([120 230 180]+128)/(256+128);patch([0 1 1 0],[0 0 1 1],c1);patch([0 1 1 1-e 1-e 0+e],[0 0 1 1-e 0+e 0+e],c2);patch([0 0 1 1-e 0+e 0+e],[0 1 1 1-e 1-e 0+e],c3);plot([0 1 1 0 0],[0 0 1 1 0]);
  mux : Mux  Inputs=1
      mask Display: e = 0.06;c1 = [120 150 230]/255;c2 = ([120 150 230]+0)/383;c3 = ([120 150 230]+128)/383;patch([0 1 1 0],[0 0 1 1],c1);patch([0 1 1 1-e 1-e 0+e],[0 0 1 1-e 0+e 0+e],c2);patch([0 0 1 1-e 0+e 0+e],[0 1 1 1-e 1-e 0+e],c3);plot([0 1 1 0 0],[0 0 1 1 0]);disp('Mux')
  "pd{2,1}" : Outport
      mask Display: e = 0.06;c1 = [120 230 180]/255;c2 = ([120 230 180]+0)/(256+128);c3 = ([120 230 180]+128)/(256+128);patch([0 1 1 0],[0 0 1 1],c1);patch([0 1 1 1-e 1-e 0+e],[0 0 1 1-e 0+e 0+e],c2);patch([0 0 1 1-e 0+e 0+e],[0 1 1 1-e 1-e 0+e],c3);plot([0 1 1 0 0],[0 0 1 1 0]);
  wires:
  "p{2}"/1 -> mux/1
  mux/1 -> "pd{2,1}"/1
